simulink model "servo_open_system"  (R2021a)
settings: Solver=VariableStepAuto  StartTime=0.0  StopTime=t_end  RelTol=1e-3
undefined symbols (not defined in the file): A, b1, b2, dt, K_sensor, Kb1, Kb2, m1, m2, mL, mM2, Ra1, Ra2, sampling, X, Y, Z
libraries: fl_lib x28, sm_lib x21, nesl_utility x14, ee_lib x7
(part 2 of 2)

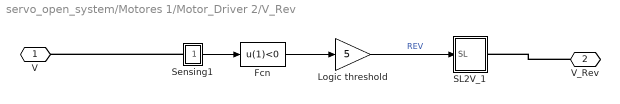
== system servo_open_system/Motores 1/Motor_Driver 2/V_Rev ==
  Fcn : Fcn  Expr=u(1)<0
  Logic threshold : Gain  Gain=5
  SL2V_1 : Subsystem
  Sensing1 : Subsystem
      mask Display: disp('V')
  V : PMIOPort  Side=Left
  V_Rev : PMIOPort  Port=2  Side=Right
  wires:
  Logic threshold/1 -> SL2V_1/1(SL)  "REV"
  Fcn/1 -> Logic threshold/1
  Sensing1/1(Out1) -> Fcn/1
  connections:
  Sensing1/LConn1 -- V/RConn1
  V_Rev/RConn1 -- SL2V_1/RConn1

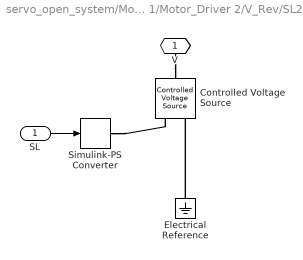
== system servo_open_system/Motores 1/Motor_Driver 2/V_Rev/SL2V_1 ==
  SL : Inport
  Controlled Voltage Source : fl_lib/Electrical/Electrical Sources/Controlled Voltage Source
  Electrical Reference : fl_lib/Electrical/Electrical Elements/Electrical Reference
  Simulink-PS Converter : nesl_utility/Simulink-PS Converter  PhysicalDomain=network_engine_domain  SubClassName=ps_input  LeftPortType=input  RightPortType=output  PseudoPeriodic=off  Frequencies=[]  NoiseDistribution=none  NoiseParameters=[]  Unit=V  AffineConversion=off  FilteringAndDerivatives=zero  SimscapeFilterOrder=1  InputFilterTimeConstant=.001  UdotUserProvided=0
      settings: SourceProductBaseCode=PW,SS
  V : PMIOPort  Side=Right
  wires:
  SL/1 -> Simulink-PS Converter/1
  connections:
  V/RConn1 -- Controlled Voltage Source/LConn1
  Simulink-PS Converter/RConn1 -- Controlled Voltage Source/RConn1
  Electrical Reference/LConn1 -- Controlled Voltage Source/RConn2

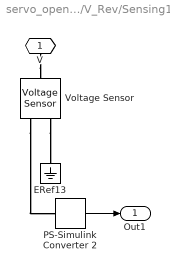
== system servo_open_system/Motores 1/Motor_Driver 2/V_Rev/Sensing1 ==
  ERef13 : fl_lib/Electrical/Electrical Elements/Electrical Reference
  PS-Simulink Converter 2 : nesl_utility/PS-Simulink Converter  PhysicalDomain=network_engine_domain  SubClassName=ps_output  LeftPortType=input  RightPortType=output  PseudoPeriodic=off  Frequencies=[]  Unit=V  AffineConversion=off
      settings: SourceProductBaseCode=PW,SS
  Voltage Sensor : fl_lib/Electrical/Electrical Sensors/Voltage Sensor
  V : PMIOPort  Side=Left
  Out1 : Outport  VectorParamsAs1DForOutWhenUnconnected=off
  wires:
  PS-Simulink Converter 2/1 -> Out1/1
  connections:
  V/RConn1 -- Voltage Sensor/LConn1
  Voltage Sensor/RConn2 -- ERef13/LConn1
  Voltage Sensor/RConn1 -- PS-Simulink Converter 2/LConn1
